simulink model "multidrivesystem"  (R2020a)
settings: Solver=ode23  StartTime=0.0  StopTime=1  MaxStep=20  RelTol=1e-4
libraries: powerlib x250
(part 2 of 2)

== system multidrivesystem/DRIVE 2 ==
  note: universal bridge rectifier
  Current Measurement : powerlib/Measurements/Current Measurement  PhasorSimulation=off  OutputType=Complex  PSBequivalent=0
  IGBT/Diode{5,8..12} (6 alike) : powerlib/Power Electronics/IGBT//Diode  Ron=1e-3  Rs=1e5  Cs=inf  Measurements=on
  Pulse Generator{6..11} (6 alike) : DiscretePulseGenerator  PulseType=Time based  Period=10  PulseWidth=5
  Scope : Scope  NumInputPorts=2
  Scopedata{9..14} (6 alike) : Scope
  Scopedata15 : Scope  NumInputPorts=2
  Series RLC Branch4 : powerlib/Elements/Series RLC Branch  LConnTagsString=__new0  RConnTagsString=__new0  BranchType=L  Resistance=1  Inductance=3e-3  SetiL0=off  InitialCurrent=0  Capacitance=1e-6  Setx0=off  InitialVoltage=0  Measurements=None
  Three-Phase Parallel RLC Load1 : powerlib/Elements/Three-Phase Parallel RLC Load  LConnTagsString=A|B|C  Configuration=Y (grounded)  NominalVoltage=1000  Vabc=[1e3 1e3 1e3]  Vabcp=[1e3 1e3 1e3]  NominalFrequency=60  UnbalancedPower=off  ActivePower=8e3  InductivePower=0  CapacitivePower=0  Pabc=[10e3 9e3 11e3]  QLabc=[100 90 110]  QCabc=[100 90 110]  Pabcp=[10e3 9e3 11e3]  QLabcp=[100 90 110]  QCabcp=[100 90 110]  Measurements=None  LoadType=constant Z
  Three-Phase V-I Measurement2 : powerlib/Measurements/Three-Phase V-I Measurement  VoltageMeasurement=phase-to-ground  SetLabelV=off  LabelV=Vabc  Vpu=off  VpuLL=off  CurrentMeasurement=yes  SetLabelI=off  LabelI=Iabc  Ipu=off  Pbase=100e6  Vbase=500e3  OutputType=Complex  PhasorSimulation=off  PSBequivalent=0
  Universal Bridge1 : powerlib/Power Electronics/Universal Bridge  Arms=3  SnubberResistance=1e5  SnubberCapacitance=inf  Device=Diodes  Ron=1e-3  Lon=0  ForwardVoltages="[  0  0  ]"  ForwardVoltage=0  GTOparameters=[ 10e-6 , 20e-6 ]  IGBTparameters=[ 1e-6 , 2e-6 ]  Measurements=None  Measurements_2=None  converterType=Rectifier
  Voltage Measurement : powerlib/Measurements/Voltage Measurement  PhasorSimulation=off  OutputType=Complex  PSBequivalent=0
  Series RLC Branch1 : PMIOPort  Side=Left
  Series RLC Branch2 : PMIOPort  Port=2  Side=Left
  Series RLC Branch3 : PMIOPort  Port=3  Side=Left
  wires:
  IGBT/Diode10/1 -> Scopedata14/1
  IGBT/Diode5/1 -> Scopedata13/1
  IGBT/Diode11/1 -> Scopedata9/1
  IGBT/Diode8/1 -> Scopedata10/1
  IGBT/Diode12/1 -> Scopedata12/1
  Pulse Generator11/1 -> IGBT/Diode12/1
  Pulse Generator8/1 -> IGBT/Diode9/1
  Three-Phase V-I Measurement2/1 -> Scopedata15/1
  Pulse Generator9/1 -> IGBT/Diode10/1
  Pulse Generator7/1 -> IGBT/Diode8/1
  Pulse Generator6/1 -> IGBT/Diode11/1
  Pulse Generator10/1 -> IGBT/Diode5/1
  Three-Phase V-I Measurement2/2 -> Scopedata15/2
  IGBT/Diode9/1 -> Scopedata11/1
  Current Measurement/1 -> Scope/1
  Voltage Measurement/1 -> Scope/2
  connections:
  Three-Phase V-I Measurement2/RConn1 -- Three-Phase Parallel RLC Load1/LConn1
  Three-Phase V-I Measurement2/RConn3 -- Three-Phase Parallel RLC Load1/LConn3
  IGBT/Diode5/LConn1 -- IGBT/Diode8/RConn1 -- Three-Phase V-I Measurement2/LConn2
  Three-Phase V-I Measurement2/RConn2 -- Three-Phase Parallel RLC Load1/LConn2
  Three-Phase V-I Measurement2/LConn1 -- IGBT/Diode11/RConn1 -- IGBT/Diode12/LConn1
  IGBT/Diode11/LConn1 -- Series RLC Branch4/RConn1 -- Voltage Measurement/LConn1 -- Current Measurement/LConn1 -- IGBT/Diode9/LConn1 -- IGBT/Diode8/LConn1
  IGBT/Diode10/LConn1 -- IGBT/Diode9/RConn1 -- Three-Phase V-I Measurement2/LConn3
  IGBT/Diode5/RConn1 -- Current Measurement/RConn1 -- Voltage Measurement/LConn2 -- Universal Bridge1/RConn2 -- IGBT/Diode12/RConn1 -- IGBT/Diode10/RConn1
  Series RLC Branch4/LConn1 -- Universal Bridge1/RConn1
  Series RLC Branch1/RConn1 -- Universal Bridge1/LConn1
  Universal Bridge1/LConn2 -- Series RLC Branch2/RConn1
  Series RLC Branch3/RConn1 -- Universal Bridge1/LConn3

== system multidrivesystem/DRIVE 20 ==
  note: universal bridge rectifier
  Current Measurement : powerlib/Measurements/Current Measurement  PhasorSimulation=off  OutputType=Complex  PSBequivalent=0
  IGBT/Diode{5,8..12} (6 alike) : powerlib/Power Electronics/IGBT//Diode  Ron=1e-3  Rs=1e5  Cs=inf  Measurements=on
  Pulse Generator{6..11} (6 alike) : DiscretePulseGenerator  PulseType=Time based  Period=10  PulseWidth=5
  Scope : Scope  NumInputPorts=2
  Scopedata{153..158} (6 alike) : Scope
  Scopedata159 : Scope  NumInputPorts=2
  Series RLC Branch4 : powerlib/Elements/Series RLC Branch  LConnTagsString=__new0  RConnTagsString=__new0  BranchType=L  Resistance=1  Inductance=3e-3  SetiL0=off  InitialCurrent=0  Capacitance=1e-6  Setx0=off  InitialVoltage=0  Measurements=None
  Three-Phase Parallel RLC Load1 : powerlib/Elements/Three-Phase Parallel RLC Load  LConnTagsString=A|B|C  Configuration=Y (grounded)  NominalVoltage=1000  Vabc=[1e3 1e3 1e3]  Vabcp=[1e3 1e3 1e3]  NominalFrequency=60  UnbalancedPower=off  ActivePower=6e3  InductivePower=0  CapacitivePower=0  Pabc=[10e3 9e3 11e3]  QLabc=[100 90 110]  QCabc=[100 90 110]  Pabcp=[10e3 9e3 11e3]  QLabcp=[100 90 110]  QCabcp=[100 90 110]  Measurements=None  LoadType=constant Z
  Three-Phase V-I Measurement2 : powerlib/Measurements/Three-Phase V-I Measurement  VoltageMeasurement=phase-to-ground  SetLabelV=off  LabelV=Vabc  Vpu=off  VpuLL=off  CurrentMeasurement=yes  SetLabelI=off  LabelI=Iabc  Ipu=off  Pbase=100e6  Vbase=500e3  OutputType=Complex  PhasorSimulation=off  PSBequivalent=0
  Universal Bridge1 : powerlib/Power Electronics/Universal Bridge  Arms=3  SnubberResistance=1e5  SnubberCapacitance=inf  Device=Diodes  Ron=1e-3  Lon=0  ForwardVoltages="[  0  0  ]"  ForwardVoltage=0  GTOparameters=[ 10e-6 , 20e-6 ]  IGBTparameters=[ 1e-6 , 2e-6 ]  Measurements=None  Measurements_2=None  converterType=Rectifier
  Voltage Measurement : powerlib/Measurements/Voltage Measurement  PhasorSimulation=off  OutputType=Complex  PSBequivalent=0
  Series RLC Branch1 : PMIOPort  Side=Left
  Series RLC Branch2 : PMIOPort  Port=2  Side=Left
  Series RLC Branch3 : PMIOPort  Port=3  Side=Left
  wires:
  IGBT/Diode10/1 -> Scopedata158/1
  IGBT/Diode5/1 -> Scopedata157/1
  IGBT/Diode11/1 -> Scopedata153/1
  IGBT/Diode8/1 -> Scopedata154/1
  IGBT/Diode12/1 -> Scopedata156/1
  Pulse Generator11/1 -> IGBT/Diode12/1
  Pulse Generator8/1 -> IGBT/Diode9/1
  Three-Phase V-I Measurement2/1 -> Scopedata159/1
  Pulse Generator9/1 -> IGBT/Diode10/1
  Pulse Generator7/1 -> IGBT/Diode8/1
  Pulse Generator6/1 -> IGBT/Diode11/1
  Pulse Generator10/1 -> IGBT/Diode5/1
  Three-Phase V-I Measurement2/2 -> Scopedata159/2
  IGBT/Diode9/1 -> Scopedata155/1
  Voltage Measurement/1 -> Scope/1
  Current Measurement/1 -> Scope/2
  connections:
  Three-Phase V-I Measurement2/RConn1 -- Three-Phase Parallel RLC Load1/LConn1
  Three-Phase V-I Measurement2/RConn3 -- Three-Phase Parallel RLC Load1/LConn3
  Three-Phase V-I Measurement2/LConn2 -- IGBT/Diode5/LConn1 -- IGBT/Diode8/RConn1
  Three-Phase V-I Measurement2/RConn2 -- Three-Phase Parallel RLC Load1/LConn2
  IGBT/Diode12/LConn1 -- Three-Phase V-I Measurement2/LConn1 -- IGBT/Diode11/RConn1
  Current Measurement/RConn1 -- IGBT/Diode12/RConn1 -- IGBT/Diode10/RConn1 -- IGBT/Diode5/RConn1 -- Voltage Measurement/LConn2 -- Universal Bridge1/RConn2
  Three-Phase V-I Measurement2/LConn3 -- IGBT/Diode10/LConn1 -- IGBT/Diode9/RConn1
  Series RLC Branch1/RConn1 -- Universal Bridge1/LConn1
  Series RLC Branch2/RConn1 -- Universal Bridge1/LConn2
  Universal Bridge1/LConn3 -- Series RLC Branch3/RConn1
  IGBT/Diode9/LConn1 -- IGBT/Diode8/LConn1 -- Series RLC Branch4/RConn1 -- Current Measurement/LConn1 -- Voltage Measurement/LConn1 -- IGBT/Diode11/LConn1
  Series RLC Branch4/LConn1 -- Universal Bridge1/RConn1

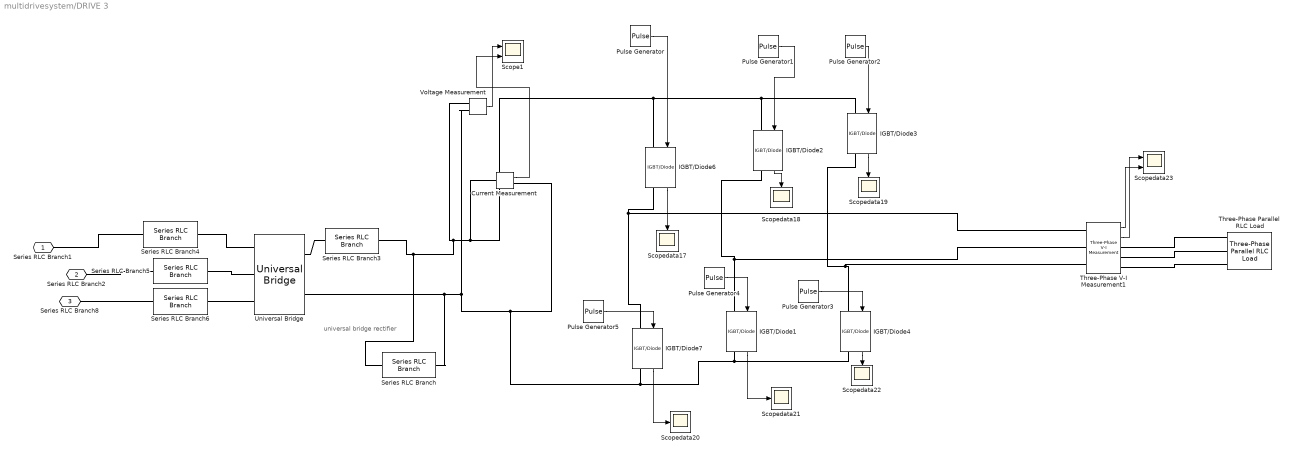
== system multidrivesystem/DRIVE 3 ==
  note: universal bridge rectifier
  Current Measurement : powerlib/Measurements/Current Measurement  PhasorSimulation=off  OutputType=Complex  PSBequivalent=0
  IGBT/Diode{1..4,6..7} (6 alike) : powerlib/Power Electronics/IGBT//Diode  Ron=1e-3  Rs=1e5  Cs=inf  Measurements=on
  Pulse Generator{,1..5} (6 alike) : DiscretePulseGenerator  PulseType=Time based  Period=10  PulseWidth=5
  Scope1 : Scope  NumInputPorts=2
  Scopedata{17..22} (6 alike) : Scope
  Scopedata23 : Scope  NumInputPorts=2
  Series RLC Branch : powerlib/Elements/Series RLC Branch  LConnTagsString=__new0  RConnTagsString=__new0  BranchType=C  Resistance=1  Inductance=1e-3  SetiL0=off  InitialCurrent=0  Capacitance=1e-6  Setx0=off  InitialVoltage=0  Measurements=None
  Series RLC Branch{3..6} (4 alike) : powerlib/Elements/Series RLC Branch  LConnTagsString=__new0  RConnTagsString=__new0  BranchType=L  Resistance=1  Inductance=3e-3  SetiL0=off  InitialCurrent=0  Capacitance=1e-6  Setx0=off  InitialVoltage=0  Measurements=None
  Three-Phase Parallel RLC Load : powerlib/Elements/Three-Phase Parallel RLC Load  LConnTagsString=A|B|C  Configuration=Y (grounded)  NominalVoltage=1000  Vabc=[1e3 1e3 1e3]  Vabcp=[1e3 1e3 1e3]  NominalFrequency=60  UnbalancedPower=off  ActivePower=10e3  InductivePower=0  CapacitivePower=0  Pabc=[10e3 9e3 11e3]  QLabc=[100 90 110]  QCabc=[100 90 110]  Pabcp=[10e3 9e3 11e3]  QLabcp=[100 90 110]  QCabcp=[100 90 110]  Measurements=None  LoadType=constant Z
  Three-Phase V-I Measurement1 : powerlib/Measurements/Three-Phase V-I Measurement  VoltageMeasurement=phase-to-ground  SetLabelV=off  LabelV=Vabc  Vpu=off  VpuLL=off  CurrentMeasurement=yes  SetLabelI=off  LabelI=Iabc  Ipu=off  Pbase=100e6  Vbase=500e3  OutputType=Complex  PhasorSimulation=off  PSBequivalent=0
  Universal Bridge : powerlib/Power Electronics/Universal Bridge  Arms=3  SnubberResistance=1e5  SnubberCapacitance=inf  Device=Diodes  Ron=1e-3  Lon=0  ForwardVoltages="[  0  0  ]"  ForwardVoltage=0  GTOparameters=[ 10e-6 , 20e-6 ]  IGBTparameters=[ 1e-6 , 2e-6 ]  Measurements=None  Measurements_2=None  converterType=Rectifier
  Voltage Measurement : powerlib/Measurements/Voltage Measurement  PhasorSimulation=off  OutputType=Complex  PSBequivalent=0
  Series RLC Branch1 : PMIOPort  Side=Left
  Series RLC Branch2 : PMIOPort  Port=2  Side=Left
  Series RLC Branch8 : PMIOPort  Port=3  Side=Left
  wires:
  IGBT/Diode1/1 -> Scopedata21/1
  IGBT/Diode3/1 -> Scopedata19/1
  Pulse Generator1/1 -> IGBT/Diode2/1
  Three-Phase V-I Measurement1/2 -> Scopedata23/1
  Pulse Generator2/1 -> IGBT/Diode3/1
  IGBT/Diode4/1 -> Scopedata22/1
  Pulse Generator5/1 -> IGBT/Diode7/1
  Pulse Generator4/1 -> IGBT/Diode1/1
  IGBT/Diode7/1 -> Scopedata20/1
  IGBT/Diode6/1 -> Scopedata17/1
  IGBT/Diode2/1 -> Scopedata18/1
  Pulse Generator/1 -> IGBT/Diode6/1
  Pulse Generator3/1 -> IGBT/Diode4/1
  Three-Phase V-I Measurement1/1 -> Scopedata23/2
  Current Measurement/1 -> Scope1/2
  Voltage Measurement/1 -> Scope1/1
  connections:
  IGBT/Diode4/LConn1 -- Three-Phase V-I Measurement1/LConn3 -- IGBT/Diode3/RConn1
  Three-Phase V-I Measurement1/RConn1 -- Three-Phase Parallel RLC Load/LConn1
  IGBT/Diode1/LConn1 -- Three-Phase V-I Measurement1/LConn2 -- IGBT/Diode2/RConn1
  Three-Phase V-I Measurement1/LConn1 -- IGBT/Diode7/LConn1 -- IGBT/Diode6/RConn1
  Three-Phase V-I Measurement1/RConn3 -- Three-Phase Parallel RLC Load/LConn3
  Three-Phase V-I Measurement1/RConn2 -- Three-Phase Parallel RLC Load/LConn2
  IGBT/Diode7/RConn1 -- Series RLC Branch/RConn1 -- Universal Bridge/RConn2 -- Voltage Measurement/LConn2 -- Current Measurement/RConn1 -- IGBT/Diode1/RConn1 -- IGBT/Diode4/RConn1
  IGBT/Diode6/LConn1 -- Series RLC Branch/LConn1 -- Series RLC Branch3/RConn1 -- Voltage Measurement/LConn1 -- Current Measurement/LConn1 -- IGBT/Diode2/LConn1 -- IGBT/Diode3/LConn1
  Series RLC Branch3/LConn1 -- Universal Bridge/RConn1
  Series RLC Branch5/LConn1 -- Series RLC Branch2/RConn1
  Series RLC Branch5/RConn1 -- Universal Bridge/LConn2
  Series RLC Branch6/LConn1 -- Series RLC Branch8/RConn1
  Series RLC Branch6/RConn1 -- Universal Bridge/LConn3
  Series RLC Branch1/RConn1 -- Series RLC Branch4/LConn1
  Series RLC Branch4/RConn1 -- Universal Bridge/LConn1

== system multidrivesystem/DRIVE 4 ==
  note: universal bridge rectifier
  Current Measurement : powerlib/Measurements/Current Measurement  PhasorSimulation=off  OutputType=Complex  PSBequivalent=0
  IGBT/Diode{1..4,6..7} (6 alike) : powerlib/Power Electronics/IGBT//Diode  Ron=1e-3  Rs=1e5  Cs=inf  Measurements=on
  Pulse Generator{,1..5} (6 alike) : DiscretePulseGenerator  PulseType=Time based  Period=10  PulseWidth=5
  Scope : Scope  NumInputPorts=2
  Scopedata{25..30} (6 alike) : Scope
  Scopedata31 : Scope  NumInputPorts=2
  Series RLC Branch3 : powerlib/Elements/Series RLC Branch  LConnTagsString=__new0  RConnTagsString=__new0  BranchType=L  Resistance=1  Inductance=3e-3  SetiL0=off  InitialCurrent=0  Capacitance=1e-6  Setx0=off  InitialVoltage=0  Measurements=None
  Three-Phase Parallel RLC Load : powerlib/Elements/Three-Phase Parallel RLC Load  LConnTagsString=A|B|C  Configuration=Y (grounded)  NominalVoltage=1000  Vabc=[1e3 1e3 1e3]  Vabcp=[1e3 1e3 1e3]  NominalFrequency=60  UnbalancedPower=off  ActivePower=4e3  InductivePower=0  CapacitivePower=0  Pabc=[10e3 9e3 11e3]  QLabc=[100 90 110]  QCabc=[100 90 110]  Pabcp=[10e3 9e3 11e3]  QLabcp=[100 90 110]  QCabcp=[100 90 110]  Measurements=None  LoadType=constant Z
  Three-Phase V-I Measurement1 : powerlib/Measurements/Three-Phase V-I Measurement  VoltageMeasurement=phase-to-ground  SetLabelV=off  LabelV=Vabc  Vpu=off  VpuLL=off  CurrentMeasurement=yes  SetLabelI=off  LabelI=Iabc  Ipu=off  Pbase=100e6  Vbase=500e3  OutputType=Complex  PhasorSimulation=off  PSBequivalent=0
  Universal Bridge : powerlib/Power Electronics/Universal Bridge  Arms=3  SnubberResistance=1e5  SnubberCapacitance=inf  Device=Diodes  Ron=1e-3  Lon=0  ForwardVoltages="[  0  0  ]"  ForwardVoltage=0  GTOparameters=[ 10e-6 , 20e-6 ]  IGBTparameters=[ 1e-6 , 2e-6 ]  Measurements=None  Measurements_2=None  converterType=Rectifier
  Voltage Measurement : powerlib/Measurements/Voltage Measurement  PhasorSimulation=off  OutputType=Complex  PSBequivalent=0
  Series RLC Branch1 : PMIOPort  Side=Left
  Series RLC Branch2 : PMIOPort  Port=2  Side=Left
  Series RLC Branch8 : PMIOPort  Port=3  Side=Left
  wires:
  Three-Phase V-I Measurement1/1 -> Scopedata31/2
  Pulse Generator3/1 -> IGBT/Diode4/1
  Pulse Generator/1 -> IGBT/Diode6/1
  IGBT/Diode2/1 -> Scopedata26/1
  IGBT/Diode6/1 -> Scopedata25/1
  IGBT/Diode7/1 -> Scopedata28/1
  Pulse Generator4/1 -> IGBT/Diode1/1
  Pulse Generator5/1 -> IGBT/Diode7/1
  IGBT/Diode4/1 -> Scopedata30/1
  Pulse Generator2/1 -> IGBT/Diode3/1
  Three-Phase V-I Measurement1/2 -> Scopedata31/1
  Pulse Generator1/1 -> IGBT/Diode2/1
  IGBT/Diode3/1 -> Scopedata27/1
  IGBT/Diode1/1 -> Scopedata29/1
  Voltage Measurement/1 -> Scope/1
  Current Measurement/1 -> Scope/2
  connections:
  Three-Phase V-I Measurement1/RConn2 -- Three-Phase Parallel RLC Load/LConn2
  Three-Phase V-I Measurement1/RConn3 -- Three-Phase Parallel RLC Load/LConn3
  IGBT/Diode6/RConn1 -- IGBT/Diode7/LConn1 -- Three-Phase V-I Measurement1/LConn1
  IGBT/Diode2/RConn1 -- Three-Phase V-I Measurement1/LConn2 -- IGBT/Diode1/LConn1
  Three-Phase V-I Measurement1/RConn1 -- Three-Phase Parallel RLC Load/LConn1
  IGBT/Diode3/RConn1 -- Three-Phase V-I Measurement1/LConn3 -- IGBT/Diode4/LConn1
  Current Measurement/RConn1 -- IGBT/Diode4/RConn1 -- IGBT/Diode1/RConn1 -- IGBT/Diode7/RConn1 -- Universal Bridge/RConn2 -- Voltage Measurement/LConn2
  Current Measurement/LConn1 -- Series RLC Branch3/RConn1 -- Voltage Measurement/LConn1 -- IGBT/Diode3/LConn1 -- IGBT/Diode2/LConn1 -- IGBT/Diode6/LConn1
  Series RLC Branch3/LConn1 -- Universal Bridge/RConn1
  Series RLC Branch1/RConn1 -- Universal Bridge/LConn1
  Series RLC Branch2/RConn1 -- Universal Bridge/LConn2
  Universal Bridge/LConn3 -- Series RLC Branch8/RConn1

== system multidrivesystem/DRIVE 5 ==
  note: universal bridge rectifier
  Current Measurement : powerlib/Measurements/Current Measurement  PhasorSimulation=off  OutputType=Complex  PSBequivalent=0
  IGBT/Diode{5,8..12} (6 alike) : powerlib/Power Electronics/IGBT//Diode  Ron=1e-3  Rs=1e5  Cs=inf  Measurements=on
  Pulse Generator{6..11} (6 alike) : DiscretePulseGenerator  PulseType=Time based  Period=10  PulseWidth=5
  Scope : Scope  NumInputPorts=2
  Scopedata{33..38} (6 alike) : Scope
  Scopedata39 : Scope  NumInputPorts=2
  Series RLC Branch4 : powerlib/Elements/Series RLC Branch  LConnTagsString=__new0  RConnTagsString=__new0  BranchType=L  Resistance=1  Inductance=3e-3  SetiL0=off  InitialCurrent=0  Capacitance=1e-6  Setx0=off  InitialVoltage=0  Measurements=None
  Three-Phase Parallel RLC Load1 : powerlib/Elements/Three-Phase Parallel RLC Load  LConnTagsString=A|B|C  Configuration=Y (grounded)  NominalVoltage=1000  Vabc=[1e3 1e3 1e3]  Vabcp=[1e3 1e3 1e3]  NominalFrequency=60  UnbalancedPower=off  ActivePower=11e3  InductivePower=0  CapacitivePower=0  Pabc=[10e3 9e3 11e3]  QLabc=[100 90 110]  QCabc=[100 90 110]  Pabcp=[10e3 9e3 11e3]  QLabcp=[100 90 110]  QCabcp=[100 90 110]  Measurements=None  LoadType=constant Z
  Three-Phase V-I Measurement2 : powerlib/Measurements/Three-Phase V-I Measurement  VoltageMeasurement=phase-to-ground  SetLabelV=off  LabelV=Vabc  Vpu=off  VpuLL=off  CurrentMeasurement=yes  SetLabelI=off  LabelI=Iabc  Ipu=off  Pbase=100e6  Vbase=500e3  OutputType=Complex  PhasorSimulation=off  PSBequivalent=0
  Universal Bridge1 : powerlib/Power Electronics/Universal Bridge  Arms=3  SnubberResistance=1e5  SnubberCapacitance=inf  Device=Diodes  Ron=1e-3  Lon=0  ForwardVoltages="[  0  0  ]"  ForwardVoltage=0  GTOparameters=[ 10e-6 , 20e-6 ]  IGBTparameters=[ 1e-6 , 2e-6 ]  Measurements=None  Measurements_2=None  converterType=Rectifier
  Voltage Measurement : powerlib/Measurements/Voltage Measurement  PhasorSimulation=off  OutputType=Complex  PSBequivalent=0
  Series RLC Branch1 : PMIOPort  Side=Left
  Series RLC Branch2 : PMIOPort  Port=2  Side=Left
  Series RLC Branch3 : PMIOPort  Port=3  Side=Left
  wires:
  IGBT/Diode9/1 -> Scopedata35/1
  Three-Phase V-I Measurement2/2 -> Scopedata39/2
  Pulse Generator10/1 -> IGBT/Diode5/1
  Pulse Generator6/1 -> IGBT/Diode11/1
  Pulse Generator7/1 -> IGBT/Diode8/1
  Pulse Generator9/1 -> IGBT/Diode10/1
  Three-Phase V-I Measurement2/1 -> Scopedata39/1
  Pulse Generator8/1 -> IGBT/Diode9/1
  Pulse Generator11/1 -> IGBT/Diode12/1
  IGBT/Diode12/1 -> Scopedata36/1
  IGBT/Diode8/1 -> Scopedata34/1
  IGBT/Diode11/1 -> Scopedata33/1
  IGBT/Diode5/1 -> Scopedata37/1
  IGBT/Diode10/1 -> Scopedata38/1
  Voltage Measurement/1 -> Scope/1
  Current Measurement/1 -> Scope/2
  connections:
  IGBT/Diode9/RConn1 -- IGBT/Diode10/LConn1 -- Three-Phase V-I Measurement2/LConn3
  IGBT/Diode11/RConn1 -- Three-Phase V-I Measurement2/LConn1 -- IGBT/Diode12/LConn1
  Three-Phase V-I Measurement2/RConn2 -- Three-Phase Parallel RLC Load1/LConn2
  IGBT/Diode8/RConn1 -- IGBT/Diode5/LConn1 -- Three-Phase V-I Measurement2/LConn2
  Three-Phase V-I Measurement2/RConn3 -- Three-Phase Parallel RLC Load1/LConn3
  Three-Phase V-I Measurement2/RConn1 -- Three-Phase Parallel RLC Load1/LConn1
  IGBT/Diode5/RConn1 -- IGBT/Diode12/RConn1 -- Current Measurement/RConn1 -- Voltage Measurement/LConn2 -- Universal Bridge1/RConn2 -- IGBT/Diode10/RConn1
  Voltage Measurement/LConn1 -- Series RLC Branch4/RConn1 -- Current Measurement/LConn1 -- IGBT/Diode11/LConn1 -- IGBT/Diode8/LConn1 -- IGBT/Diode9/LConn1
  Series RLC Branch4/LConn1 -- Universal Bridge1/RConn1
  Series RLC Branch1/RConn1 -- Universal Bridge1/LConn1
  Series RLC Branch2/RConn1 -- Universal Bridge1/LConn2
  Universal Bridge1/LConn3 -- Series RLC Branch3/RConn1

== system multidrivesystem/DRIVE 6 ==
  note: universal bridge rectifier
  Current Measurement : powerlib/Measurements/Current Measurement  PhasorSimulation=off  OutputType=Complex  PSBequivalent=0
  IGBT/Diode{5,8..12} (6 alike) : powerlib/Power Electronics/IGBT//Diode  Ron=1e-3  Rs=1e5  Cs=inf  Measurements=on
  Pulse Generator{6..11} (6 alike) : DiscretePulseGenerator  PulseType=Time based  Period=10  PulseWidth=5
  Scope1 : Scope  NumInputPorts=2
  Scopedata{41..46} (6 alike) : Scope
  Scopedata47 : Scope  NumInputPorts=2
  Series RLC Branch4 : powerlib/Elements/Series RLC Branch  LConnTagsString=__new0  RConnTagsString=__new0  BranchType=L  Resistance=1  Inductance=3e-3  SetiL0=off  InitialCurrent=0  Capacitance=1e-6  Setx0=off  InitialVoltage=0  Measurements=None
  Three-Phase Parallel RLC Load1 : powerlib/Elements/Three-Phase Parallel RLC Load  LConnTagsString=A|B|C  Configuration=Y (grounded)  NominalVoltage=1000  Vabc=[1e3 1e3 1e3]  Vabcp=[1e3 1e3 1e3]  NominalFrequency=60  UnbalancedPower=off  ActivePower=8e3  InductivePower=0  CapacitivePower=0  Pabc=[10e3 9e3 11e3]  QLabc=[100 90 110]  QCabc=[100 90 110]  Pabcp=[10e3 9e3 11e3]  QLabcp=[100 90 110]  QCabcp=[100 90 110]  Measurements=None  LoadType=constant Z
  Three-Phase V-I Measurement2 : powerlib/Measurements/Three-Phase V-I Measurement  VoltageMeasurement=phase-to-ground  SetLabelV=off  LabelV=Vabc  Vpu=off  VpuLL=off  CurrentMeasurement=yes  SetLabelI=off  LabelI=Iabc  Ipu=off  Pbase=100e6  Vbase=500e3  OutputType=Complex  PhasorSimulation=off  PSBequivalent=0
  Universal Bridge1 : powerlib/Power Electronics/Universal Bridge  Arms=3  SnubberResistance=1e5  SnubberCapacitance=inf  Device=Diodes  Ron=1e-3  Lon=0  ForwardVoltages="[  0  0  ]"  ForwardVoltage=0  GTOparameters=[ 10e-6 , 20e-6 ]  IGBTparameters=[ 1e-6 , 2e-6 ]  Measurements=None  Measurements_2=None  converterType=Rectifier
  Voltage Measurement : powerlib/Measurements/Voltage Measurement  PhasorSimulation=off  OutputType=Complex  PSBequivalent=0
  Series RLC Branch1 : PMIOPort  Side=Left
  Series RLC Branch2 : PMIOPort  Port=2  Side=Left
  Series RLC Branch3 : PMIOPort  Port=3  Side=Left
  wires:
  IGBT/Diode10/1 -> Scopedata46/1
  IGBT/Diode5/1 -> Scopedata45/1
  IGBT/Diode11/1 -> Scopedata41/1
  IGBT/Diode8/1 -> Scopedata42/1
  IGBT/Diode12/1 -> Scopedata44/1
  Pulse Generator11/1 -> IGBT/Diode12/1
  Pulse Generator8/1 -> IGBT/Diode9/1
  Three-Phase V-I Measurement2/1 -> Scopedata47/1
  Pulse Generator9/1 -> IGBT/Diode10/1
  Pulse Generator7/1 -> IGBT/Diode8/1
  Pulse Generator6/1 -> IGBT/Diode11/1
  Pulse Generator10/1 -> IGBT/Diode5/1
  Three-Phase V-I Measurement2/2 -> Scopedata47/2
  IGBT/Diode9/1 -> Scopedata43/1
  Current Measurement/1 -> Scope1/2
  Voltage Measurement/1 -> Scope1/1
  connections:
  Three-Phase V-I Measurement2/RConn1 -- Three-Phase Parallel RLC Load1/LConn1
  Three-Phase V-I Measurement2/RConn3 -- Three-Phase Parallel RLC Load1/LConn3
  Three-Phase V-I Measurement2/LConn2 -- IGBT/Diode5/LConn1 -- IGBT/Diode8/RConn1
  Three-Phase V-I Measurement2/RConn2 -- Three-Phase Parallel RLC Load1/LConn2
  IGBT/Diode12/LConn1 -- Three-Phase V-I Measurement2/LConn1 -- IGBT/Diode11/RConn1
  Voltage Measurement/LConn1 -- Series RLC Branch4/RConn1 -- Current Measurement/LConn1 -- IGBT/Diode9/LConn1 -- IGBT/Diode8/LConn1 -- IGBT/Diode11/LConn1
  Three-Phase V-I Measurement2/LConn3 -- IGBT/Diode10/LConn1 -- IGBT/Diode9/RConn1
  IGBT/Diode10/RConn1 -- Voltage Measurement/LConn2 -- Universal Bridge1/RConn2 -- Current Measurement/RConn1 -- IGBT/Diode12/RConn1 -- IGBT/Diode5/RConn1
  Series RLC Branch4/LConn1 -- Universal Bridge1/RConn1
  Series RLC Branch1/RConn1 -- Universal Bridge1/LConn1
  Series RLC Branch2/RConn1 -- Universal Bridge1/LConn2
  Universal Bridge1/LConn3 -- Series RLC Branch3/RConn1

== system multidrivesystem/DRIVE 7  ==
  note: universal bridge rectifier
  Current Measurement : powerlib/Measurements/Current Measurement  PhasorSimulation=off  OutputType=Complex  PSBequivalent=0
  IGBT/Diode{5,8..12} (6 alike) : powerlib/Power Electronics/IGBT//Diode  Ron=1e-3  Rs=1e5  Cs=inf  Measurements=on
  Pulse Generator{6..11} (6 alike) : DiscretePulseGenerator  PulseType=Time based  Period=10  PulseWidth=5
  Scope : Scope  NumInputPorts=2
  Scopedata{49..51,54..56} (6 alike) : Scope
  Scopedata52 : Scope  NumInputPorts=2
  Series RLC Branch4 : powerlib/Elements/Series RLC Branch  LConnTagsString=__new0  RConnTagsString=__new0  BranchType=L  Resistance=1  Inductance=3e-3  SetiL0=off  InitialCurrent=0  Capacitance=1e-6  Setx0=off  InitialVoltage=0  Measurements=None
  Three-Phase Parallel RLC Load1 : powerlib/Elements/Three-Phase Parallel RLC Load  LConnTagsString=A|B|C  Configuration=Y (grounded)  NominalVoltage=1000  Vabc=[1e3 1e3 1e3]  Vabcp=[1e3 1e3 1e3]  NominalFrequency=60  UnbalancedPower=off  ActivePower=12e3  InductivePower=0  CapacitivePower=0  Pabc=[10e3 9e3 11e3]  QLabc=[100 90 110]  QCabc=[100 90 110]  Pabcp=[10e3 9e3 11e3]  QLabcp=[100 90 110]  QCabcp=[100 90 110]  Measurements=None  LoadType=constant Z
  Three-Phase V-I Measurement2 : powerlib/Measurements/Three-Phase V-I Measurement  VoltageMeasurement=phase-to-ground  SetLabelV=off  LabelV=Vabc  Vpu=off  VpuLL=off  CurrentMeasurement=yes  SetLabelI=off  LabelI=Iabc  Ipu=off  Pbase=100e6  Vbase=500e3  OutputType=Complex  PhasorSimulation=off  PSBequivalent=0
  Universal Bridge1 : powerlib/Power Electronics/Universal Bridge  Arms=3  SnubberResistance=1e5  SnubberCapacitance=inf  Device=Diodes  Ron=1e-3  Lon=0  ForwardVoltages="[  0  0  ]"  ForwardVoltage=0  GTOparameters=[ 10e-6 , 20e-6 ]  IGBTparameters=[ 1e-6 , 2e-6 ]  Measurements=None  Measurements_2=None  converterType=Rectifier
  Voltage Measurement : powerlib/Measurements/Voltage Measurement  PhasorSimulation=off  OutputType=Complex  PSBequivalent=0
  Series RLC Branch1 : PMIOPort  Side=Left
  Series RLC Branch2 : PMIOPort  Port=2  Side=Left
  Series RLC Branch3 : PMIOPort  Port=3  Side=Left
  wires:
  IGBT/Diode10/1 -> Scopedata56/1
  IGBT/Diode5/1 -> Scopedata55/1
  IGBT/Diode11/1 -> Scopedata49/1
  IGBT/Diode8/1 -> Scopedata50/1
  IGBT/Diode12/1 -> Scopedata54/1
  Pulse Generator11/1 -> IGBT/Diode12/1
  Pulse Generator8/1 -> IGBT/Diode9/1
  Three-Phase V-I Measurement2/1 -> Scopedata52/1
  Pulse Generator9/1 -> IGBT/Diode10/1
  Pulse Generator7/1 -> IGBT/Diode8/1
  Pulse Generator6/1 -> IGBT/Diode11/1
  Pulse Generator10/1 -> IGBT/Diode5/1
  Three-Phase V-I Measurement2/2 -> Scopedata52/2
  IGBT/Diode9/1 -> Scopedata51/1
  Voltage Measurement/1 -> Scope/2
  Current Measurement/1 -> Scope/1
  connections:
  Three-Phase V-I Measurement2/RConn1 -- Three-Phase Parallel RLC Load1/LConn1
  Three-Phase V-I Measurement2/RConn3 -- Three-Phase Parallel RLC Load1/LConn3
  Three-Phase V-I Measurement2/LConn2 -- IGBT/Diode5/LConn1 -- IGBT/Diode8/RConn1
  Three-Phase V-I Measurement2/RConn2 -- Three-Phase Parallel RLC Load1/LConn2
  IGBT/Diode12/LConn1 -- Three-Phase V-I Measurement2/LConn1 -- IGBT/Diode11/RConn1
  Three-Phase V-I Measurement2/LConn3 -- IGBT/Diode10/LConn1 -- IGBT/Diode9/RConn1
  IGBT/Diode5/RConn1 -- Current Measurement/RConn1 -- Voltage Measurement/LConn2 -- Universal Bridge1/RConn2 -- IGBT/Diode12/RConn1 -- IGBT/Diode10/RConn1
  IGBT/Diode9/LConn1 -- IGBT/Diode8/LConn1 -- Series RLC Branch4/RConn1 -- Current Measurement/LConn1 -- Voltage Measurement/LConn1 -- IGBT/Diode11/LConn1
  Series RLC Branch4/LConn1 -- Universal Bridge1/RConn1
  Series RLC Branch1/RConn1 -- Universal Bridge1/LConn1
  Universal Bridge1/LConn2 -- Series RLC Branch2/RConn1
  Series RLC Branch3/RConn1 -- Universal Bridge1/LConn3

== system multidrivesystem/DRIVE 8 ==
  note: universal bridge rectifier
  Current Measurement : powerlib/Measurements/Current Measurement  PhasorSimulation=off  OutputType=Complex  PSBequivalent=0
  IGBT/Diode{5,8..12} (6 alike) : powerlib/Power Electronics/IGBT//Diode  Ron=1e-3  Rs=1e5  Cs=inf  Measurements=on
  Pulse Generator{6..11} (6 alike) : DiscretePulseGenerator  PulseType=Time based  Period=10  PulseWidth=5
  Scope : Scope  NumInputPorts=2
  Scopedata{57..62} (6 alike) : Scope
  Scopedata63 : Scope  NumInputPorts=2
  Series RLC Branch4 : powerlib/Elements/Series RLC Branch  LConnTagsString=__new0  RConnTagsString=__new0  BranchType=L  Resistance=1  Inductance=3e-3  SetiL0=off  InitialCurrent=0  Capacitance=1e-6  Setx0=off  InitialVoltage=0  Measurements=None
  Three-Phase Parallel RLC Load1 : powerlib/Elements/Three-Phase Parallel RLC Load  LConnTagsString=A|B|C  Configuration=Y (grounded)  NominalVoltage=1000  Vabc=[1e3 1e3 1e3]  Vabcp=[1e3 1e3 1e3]  NominalFrequency=60  UnbalancedPower=off  ActivePower=3e3  InductivePower=0  CapacitivePower=0  Pabc=[10e3 9e3 11e3]  QLabc=[100 90 110]  QCabc=[100 90 110]  Pabcp=[10e3 9e3 11e3]  QLabcp=[100 90 110]  QCabcp=[100 90 110]  Measurements=None  LoadType=constant Z
  Three-Phase V-I Measurement2 : powerlib/Measurements/Three-Phase V-I Measurement  VoltageMeasurement=phase-to-ground  SetLabelV=off  LabelV=Vabc  Vpu=off  VpuLL=off  CurrentMeasurement=yes  SetLabelI=off  LabelI=Iabc  Ipu=off  Pbase=100e6  Vbase=500e3  OutputType=Complex  PhasorSimulation=off  PSBequivalent=0
  Universal Bridge1 : powerlib/Power Electronics/Universal Bridge  Arms=3  SnubberResistance=1e5  SnubberCapacitance=inf  Device=Diodes  Ron=1e-3  Lon=0  ForwardVoltages="[  0  0  ]"  ForwardVoltage=0  GTOparameters=[ 10e-6 , 20e-6 ]  IGBTparameters=[ 1e-6 , 2e-6 ]  Measurements=None  Measurements_2=None  converterType=Rectifier
  Voltage Measurement : powerlib/Measurements/Voltage Measurement  PhasorSimulation=off  OutputType=Complex  PSBequivalent=0
  Series RLC Branch1 : PMIOPort  Side=Left
  Series RLC Branch2 : PMIOPort  Port=2  Side=Left
  Series RLC Branch3 : PMIOPort  Port=3  Side=Left
  wires:
  IGBT/Diode9/1 -> Scopedata59/1
  Three-Phase V-I Measurement2/2 -> Scopedata63/2
  Pulse Generator10/1 -> IGBT/Diode5/1
  Pulse Generator6/1 -> IGBT/Diode11/1
  Pulse Generator7/1 -> IGBT/Diode8/1
  Pulse Generator9/1 -> IGBT/Diode10/1
  Three-Phase V-I Measurement2/1 -> Scopedata63/1
  Pulse Generator8/1 -> IGBT/Diode9/1
  Pulse Generator11/1 -> IGBT/Diode12/1
  IGBT/Diode12/1 -> Scopedata60/1
  IGBT/Diode8/1 -> Scopedata58/1
  IGBT/Diode11/1 -> Scopedata57/1
  IGBT/Diode5/1 -> Scopedata61/1
  IGBT/Diode10/1 -> Scopedata62/1
  Voltage Measurement/1 -> Scope/1
  Current Measurement/1 -> Scope/2
  connections:
  IGBT/Diode9/RConn1 -- IGBT/Diode10/LConn1 -- Three-Phase V-I Measurement2/LConn3
  IGBT/Diode5/RConn1 -- IGBT/Diode10/RConn1 -- IGBT/Diode12/RConn1 -- Current Measurement/RConn1 -- Voltage Measurement/LConn2 -- Universal Bridge1/RConn2
  IGBT/Diode11/RConn1 -- Three-Phase V-I Measurement2/LConn1 -- IGBT/Diode12/LConn1
  Three-Phase V-I Measurement2/RConn2 -- Three-Phase Parallel RLC Load1/LConn2
  Voltage Measurement/LConn1 -- Series RLC Branch4/RConn1 -- Current Measurement/LConn1 -- IGBT/Diode11/LConn1 -- IGBT/Diode8/LConn1 -- IGBT/Diode9/LConn1
  IGBT/Diode8/RConn1 -- IGBT/Diode5/LConn1 -- Three-Phase V-I Measurement2/LConn2
  Three-Phase V-I Measurement2/RConn3 -- Three-Phase Parallel RLC Load1/LConn3
  Three-Phase V-I Measurement2/RConn1 -- Three-Phase Parallel RLC Load1/LConn1
  Universal Bridge1/RConn1 -- Series RLC Branch4/LConn1
  Series RLC Branch1/RConn1 -- Universal Bridge1/LConn1
  Series RLC Branch2/RConn1 -- Universal Bridge1/LConn2
  Series RLC Branch3/RConn1 -- Universal Bridge1/LConn3

== system multidrivesystem/DRIVE 9 ==
  note: universal bridge rectifier
  Current Measurement : powerlib/Measurements/Current Measurement  PhasorSimulation=off  OutputType=Complex  PSBequivalent=0
  IGBT/Diode{5,8..12} (6 alike) : powerlib/Power Electronics/IGBT//Diode  Ron=1e-3  Rs=1e5  Cs=inf  Measurements=on
  Pulse Generator{6..11} (6 alike) : DiscretePulseGenerator  PulseType=Time based  Period=10  PulseWidth=5
  Scope : Scope  NumInputPorts=2
  Scopedata{65..70} (6 alike) : Scope
  Scopedata71 : Scope  NumInputPorts=2
  Series RLC Branch4 : powerlib/Elements/Series RLC Branch  LConnTagsString=__new0  RConnTagsString=__new0  BranchType=L  Resistance=1  Inductance=3e-3  SetiL0=off  InitialCurrent=0  Capacitance=1e-6  Setx0=off  InitialVoltage=0  Measurements=None
  Three-Phase Parallel RLC Load1 : powerlib/Elements/Three-Phase Parallel RLC Load  LConnTagsString=A|B|C  Configuration=Y (grounded)  NominalVoltage=1000  Vabc=[1e3 1e3 1e3]  Vabcp=[1e3 1e3 1e3]  NominalFrequency=60  UnbalancedPower=off  ActivePower=7e3  InductivePower=0  CapacitivePower=0  Pabc=[10e3 9e3 11e3]  QLabc=[100 90 110]  QCabc=[100 90 110]  Pabcp=[10e3 9e3 11e3]  QLabcp=[100 90 110]  QCabcp=[100 90 110]  Measurements=None  LoadType=constant Z
  Three-Phase V-I Measurement2 : powerlib/Measurements/Three-Phase V-I Measurement  VoltageMeasurement=phase-to-ground  SetLabelV=off  LabelV=Vabc  Vpu=off  VpuLL=off  CurrentMeasurement=yes  SetLabelI=off  LabelI=Iabc  Ipu=off  Pbase=100e6  Vbase=500e3  OutputType=Complex  PhasorSimulation=off  PSBequivalent=0
  Universal Bridge1 : powerlib/Power Electronics/Universal Bridge  Arms=3  SnubberResistance=1e5  SnubberCapacitance=inf  Device=Diodes  Ron=1e-3  Lon=0  ForwardVoltages="[  0  0  ]"  ForwardVoltage=0  GTOparameters=[ 10e-6 , 20e-6 ]  IGBTparameters=[ 1e-6 , 2e-6 ]  Measurements=None  Measurements_2=None  converterType=Rectifier
  Voltage Measurement : powerlib/Measurements/Voltage Measurement  PhasorSimulation=off  OutputType=Complex  PSBequivalent=0
  Series RLC Branch1 : PMIOPort  Side=Left
  Series RLC Branch2 : PMIOPort  Port=2  Side=Left
  Series RLC Branch3 : PMIOPort  Port=3  Side=Left
  wires:
  IGBT/Diode9/1 -> Scopedata67/1
  Three-Phase V-I Measurement2/2 -> Scopedata71/1
  Pulse Generator10/1 -> IGBT/Diode5/1
  Pulse Generator6/1 -> IGBT/Diode11/1
  Pulse Generator7/1 -> IGBT/Diode8/1
  Pulse Generator9/1 -> IGBT/Diode10/1
  Three-Phase V-I Measurement2/1 -> Scopedata71/2
  Pulse Generator8/1 -> IGBT/Diode9/1
  Pulse Generator11/1 -> IGBT/Diode12/1
  IGBT/Diode12/1 -> Scopedata68/1
  IGBT/Diode8/1 -> Scopedata66/1
  IGBT/Diode11/1 -> Scopedata65/1
  IGBT/Diode5/1 -> Scopedata69/1
  IGBT/Diode10/1 -> Scopedata70/1
  Voltage Measurement/1 -> Scope/2
  Current Measurement/1 -> Scope/1
  connections:
  Voltage Measurement/LConn1 -- Series RLC Branch4/RConn1 -- Current Measurement/LConn1 -- IGBT/Diode11/LConn1 -- IGBT/Diode8/LConn1 -- IGBT/Diode9/LConn1
  IGBT/Diode9/RConn1 -- IGBT/Diode10/LConn1 -- Three-Phase V-I Measurement2/LConn3
  IGBT/Diode5/RConn1 -- IGBT/Diode10/RConn1 -- IGBT/Diode12/RConn1 -- Current Measurement/RConn1 -- Voltage Measurement/LConn2 -- Universal Bridge1/RConn2
  IGBT/Diode11/RConn1 -- Three-Phase V-I Measurement2/LConn1 -- IGBT/Diode12/LConn1
  Three-Phase V-I Measurement2/RConn2 -- Three-Phase Parallel RLC Load1/LConn2
  IGBT/Diode8/RConn1 -- IGBT/Diode5/LConn1 -- Three-Phase V-I Measurement2/LConn2
  Three-Phase V-I Measurement2/RConn3 -- Three-Phase Parallel RLC Load1/LConn3
  Three-Phase V-I Measurement2/RConn1 -- Three-Phase Parallel RLC Load1/LConn1
  Series RLC Branch4/LConn1 -- Universal Bridge1/RConn1
  Universal Bridge1/LConn1 -- Series RLC Branch1/RConn1
  Universal Bridge1/LConn2 -- Series RLC Branch2/RConn1
  Universal Bridge1/LConn3 -- Series RLC Branch3/RConn1
